simulink model "turnlamp"  (R2016a)
settings: Solver=ode1  StartTime=0.0  StopTime=Inf  FixedStep=0.001  RelTol=1e-3
PostLoadFcn:
  | , if any(exist('dsrtsu_mdlpostloadfcn', 'file') == [2, 3, 6]), try dsrtsu_mdlpostloadfcn('Execute', bdroot); catch fprintf('Error in PostLoadFcn (dsrtsu_mdlpostloadfcn) for model "%s":\n %s\n', bdroot, lasterr); end, end,
  | 
  | % Begin Version: 1.0
  | if(3 == exist('DSWatchDog')), DSWatchDog('OpenModel', get_param(bdroot(gcs),'filename')); end; assignin('base', sprintf('DS_%s_STATE', upper(bdroot(gcs))), 0);
  | % End Version: 1.0
StartFcn:
  | % Begin Version: 1.0
  | if(3 == exist('DSWatchDog')), DSWatchDog('StartModel', get_param(bdroot(gcs),'filename')); end; assignin('base', sprintf('DS_%s_STATE', upper(bdroot(gcs))), 2);
  | % End Version: 1.0
StopFcn:
  | % Begin Version: 1.0
  | if(3 == exist('DSWatchDog')), DSWatchDog('StopModel', get_param(bdroot(gcs),'filename')); end; assignin('base', sprintf('DS_%s_STATE', upper(bdroot(gcs))), 0);
  | % End Version: 1.0
libraries: simulink x2, simulink_extras x2
PreSaveFcn:
  | % Begin Version: 1.0
  | OldName = get_param(bdroot(gcs), 'Tag'); NewName = get_param(bdroot(gcs), 'filename'); if (~strcmp(OldName, NewName)), if(3 == exist('DSWatchDog')), DSWatchDog('CloseModel', OldName); DSWatchDog('OpenModel', NewName); end; set_param(bdroot(gcs), 'Tag', NewName); end; try, evalin('base', 'clear OldName NewName'); catch, disp('Error during execution of PreSaveFcn callback'); end;
  | % End Version: 1.0
PostSaveFcn:
  | % Begin Version: 1.0
  | if(3 == exist('DSWatchDog')), DSWatchDog('SaveModel', get_param(bdroot(gcs),'filename')); end;
  | % End Version: 1.0
CloseFcn:
  | % Begin Version: 1.0
  | if(3 == exist('DSWatchDog')), DSWatchDog('CloseModel', get_param(bdroot(gcs),'filename')); end; try, DS_STATE_NAME = sprintf('DS_%s_STATE', upper(bdroot(gcs))); evalin('base', 'clear(DS_STATE_NAME)'); evalin('base', 'clear DS_STATE_NAME'); catch, disp('Error during execution of CloseFcn callback'); end;
  | % End Version: 1.0
settings Model: Tag=C:\Users\Admin\Documents\dSPACE\Real-Time Testing\3.3\SampleExperiments\TurnSignal_VEOS\Model\turnlamp.slx  RTICANMMDATA=struct('GeneralSetupData',struct('modelroot',['C:\Users\Admin\Documents\dSPACE\Real-Time Testing\2.6\SampleExperiments\TurnSignal_VEOS\Model'],'generalsettings',struct('filesettings',struct('destfolder',struct('Name','RTICANMM_FILES','Check',1),'buildfolder',struct('Name','.','Check',1),'AbsDestfolder',struct('Name',['C:\Users\Admin\Documents\dSPACE\Real-Time Testing\2.6\SampleExperiments\TurnSignal_VEOS\Model\RTICANMM_FILES']),'AbsBuildfolder',struct('Name',['C:\Users\Admin\Documents\dSPACE\Real-Time Testing\2.6\SampleExperiments\TurnSignal_VEOS\Model']))),'options',struct('addpaths',1,'rmpaths',1,'addtrcexclusion',logical(1),'cannavigator',struct('checkmonitoring',0),'show_usrtrc',0,'use_usrtrc',0),'advanced',struct('options',[1 1 1 1 1 1 1 1 1 1 1 1 1 1 1 1 1 1 1 1 1 1 1 1 1 1 1 1 1 1 1 1 1 1 1 1 1 1 1 1 1 1 1 1 1 1 1 1 1 1 1 1 1 1 1 1 1 1 1 1 1 1 1 1 1 1 1 1 1 1 1 1 1 1 1 1 1 1 1 1 1 1 1 1 1 1 1 1 1 1 1 1 1 1 1 1 1 1 1 1]),'MPSetup',{{}},'modelname','turnlamp','block','turnlamp'))  RTILINMMDATA=struct('GeneralSetupData',[])  DSRTSU_INTERNAL_RTI_VER=460  DSRTSU_INTERNAL_RTI_TYPE=rti1401  DSRTSU_INTERNAL_RTIFLEXRAYCONFIG=80  DSRTSU_INTERNAL_RTIFPGA=50  ModifiedByFormat=dSPACE GmbH  ExtModeTrigMode=oneshot  ExtModeArmWhenConnect=off  Creator=dSPACE GmbH  LastModifiedBy=dSPACE GmbH
settings DataIOCC: LimitDataPoints=on  SaveFormat=Array  SignalLoggingSaveFormat=ModelDataLogs
settings OptimizationCC: BlockReduction=off  ConditionallyExecuteInputs=off  OptimizeBlockIOStorage=off  BufferReuse=off  GlobalBufferReuse=off  ExpressionFolding=off  ExpressionDepthLimit=2147483647  LocalBlockOutputs=off  InitFltsAndDblsToZero=on
settings DebuggingCC: SaveWithParameterizedLinksMsg=none  UnderspecifiedInitializationDetection=Classic  MergeDetectMultiDrivingBlocksExec=none  SignalResolutionControl=TryResolveAllWithWarning  MultiTaskDSMMsg=warning  MultiTaskCondExecSysMsg=none  MultiTaskRateTransMsg=warning  FcnCallInpInsideContextMsg=UseLocalSettings  StateNameClashWarn=warning
settings HardwareCC: ProdBitPerPointer=32  ProdLargestAtomicFloat=None  ProdIntDivRoundTo=Undefined  ProdEndianess=Unspecified  ProdWordSize=32  ProdHWDeviceType=32-bit Generic  TargetIntDivRoundTo=Zero  TargetEndianess=BigEndian  TargetHWDeviceType=Generic->Custom
settings ModelReferenceCC: PropagateSignalLabelsOutOfModel=off
settings RTWCC: SystemTargetFile=dsrt.tlc  GenCodeOnly=on  MakeCommand=make_dsrt  TemplateMakefile=dsrt_default_tmf  Description=dSPACE Run-Time Target  RTWVerbose=off
settings STFCustomTargetCC: ParMdlRefBuildCompliant=on  GeneratePreprocessorConditionals=Disable all  SystemTargetFile=dsrt.tlc
settings GRTTargetCC: CompOptLevelCompliant=off  ConcurrentExecutionCompliant=off  CombineOutputUpdateFcns=off  MatFileLogging=off  CPPClassGenCompliant=off  GRTInterface=on  UseToolchainInfoCompliant=off
settings ConfigComp: CovModelRefEnable=Off  CovSFcnEnable=off

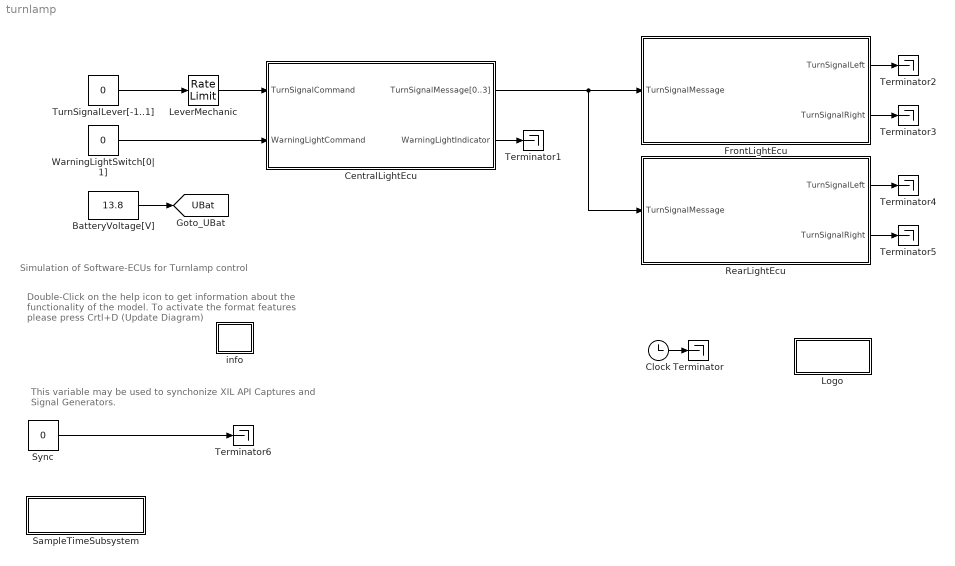
== system turnlamp ==
  note: This variable may be used to synchonize XIL API Captures
      | and Signal Generators.
  note: Simulation of Software-ECUs for Turnlamp control
  note: Double-Click on the help icon to get information about
      | the functionality of the model.
      |
      | To activate the format features please
      | press Crtl+D (Update Diagram)
  BatteryVoltage[V] : Constant  Value=13.8
  CentralLightEcu : Subsystem
  Clock : Clock
  FrontLightEcu : Subsystem
  LeverMechanic : RateLimiter  RisingSlewLimit=25  FallingSlewLimit=-25
  Logo : Subsystem  mask(dSPACE){EmptyParameter=[]}
      mask prompts: EmptyParameter "Mask Parameter 1:"
      settings: OpenFcn=;
      mask Display: image(imread('rti_mdl_dslogo.tif'));
  RearLightEcu : Subsystem
  SampleTimeSubsystem : Subsystem  TreatAsAtomicUnit=on  SystemSampleTime=0.01
  Sync : Constant  Value=0
  Terminator{,1..6} (7 alike) : Terminator
  TurnSignalLever[-1..1] : Constant  Value=0
  WarningLightSwitch[0|1] : Constant  Value=0
  info : Subsystem
      mask Display: disp('?')
  tag scope: UBat=global
  wires:
  TurnSignalLever[-1..1]/1 -> LeverMechanic/1
  LeverMechanic/1 -> CentralLightEcu/1(TurnSignalCommand)
  WarningLightSwitch[0|1]/1 -> CentralLightEcu/2(WarningLightCommand)
  CentralLightEcu/1(TurnSignalMessage[0..3]) -> FrontLightEcu/1(TurnSignalMessage), RearLightEcu/1(TurnSignalMessage)
  CentralLightEcu/2(WarningLightIndicator) -> Terminator1/1
  BatteryVoltage[V]/1 -> [UBat]
  FrontLightEcu/1(TurnSignalLeft) -> Terminator2/1
  FrontLightEcu/2(TurnSignalRight) -> Terminator3/1
  RearLightEcu/1(TurnSignalLeft) -> Terminator4/1
  RearLightEcu/2(TurnSignalRight) -> Terminator5/1
  Clock/1 -> Terminator/1
  Sync/1 -> Terminator6/1

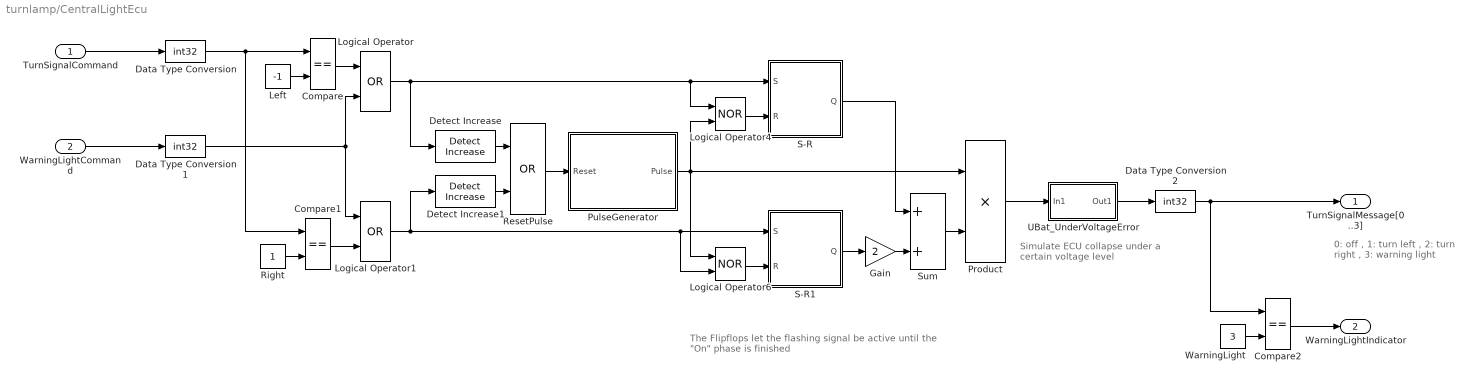
== system turnlamp/CentralLightEcu ==
  note: 0: off               ,
      | 1: turn left       ,
      | 2: turn right     ,
      | 3: warning light
  note: Simulate ECU collapse
      | under a certain voltage level
  note: The Flipflops let the flashing signal be active until
      | the "On" phase is finished
  TurnSignalCommand : Inport
  WarningLightCommand : Inport  Port=2
  Compare : RelationalOperator  Operator===  OutDataTypeStr=uint(8)  ZeroCross=off  InputSameDT=on
  Compare1 : RelationalOperator  Operator===  OutDataTypeStr=uint(8)  ZeroCross=off  InputSameDT=on
  Compare2 : RelationalOperator  Operator===  OutDataTypeStr=uint(8)  ZeroCross=off  InputSameDT=on
  Data Type Conversion : DataTypeConversion  OutDataTypeStr=int32  RndMeth=Zero
  Data Type Conversion1 : DataTypeConversion  OutDataTypeStr=int32  RndMeth=Zero
  Data Type Conversion2 : DataTypeConversion  OutDataTypeStr=int32  RndMeth=Zero
  Detect Increase : simulink/Logic and Bit Operations/Detect Increase  vinit=0.0  InputProcessing=Inherited  OutDataTypeStr=boolean
  Detect Increase1 : simulink/Logic and Bit Operations/Detect Increase  vinit=0.0  InputProcessing=Inherited  OutDataTypeStr=boolean
  Gain : Gain  Gain=2
  Left : Constant  Value=-1  OutDataTypeStr=Inherit: Inherit via back propagation
  Logical Operator : Logic  Operator=OR  AllPortsSameDT=off  OutDataTypeStr=uint(8)
  Logical Operator1 : Logic  Operator=OR  AllPortsSameDT=off  OutDataTypeStr=uint(8)
  Logical Operator4 : Logic  Operator=NOR  AllPortsSameDT=off  OutDataTypeStr=uint(8)
  Logical Operator6 : Logic  Operator=NOR  AllPortsSameDT=off  OutDataTypeStr=uint(8)
  Product : Product  RndMeth=Zero
  PulseGenerator : Subsystem
  ResetPulse : Logic  Operator=OR  AllPortsSameDT=off  OutDataTypeStr=uint(8)
  Right : Constant  OutDataTypeStr=Inherit: Inherit via back propagation
  S-R : Subsystem
  S-R1 : Subsystem
  Sum : Sum
  UBat_UnderVoltageError : Subsystem
  WarningLight : Constant  Value=3  OutDataTypeStr=Inherit: Inherit via back propagation
  TurnSignalMessage[0..3] : Outport
  WarningLightIndicator : Outport  Port=2
  wires:
  Data Type Conversion/1 -> Compare/1, Compare1/1
  Compare/1 -> Logical Operator/1
  Data Type Conversion1/1 -> Logical Operator/2, Logical Operator1/1
  Compare1/1 -> Logical Operator1/2
  Gain/1 -> Sum/2
  TurnSignalCommand/1 -> Data Type Conversion/1
  Product/1 -> UBat_UnderVoltageError/1(In1)
  WarningLightCommand/1 -> Data Type Conversion1/1
  Compare2/1 -> WarningLightIndicator/1
  Logical Operator/1 -> Logical Operator4/1, S-R/1(S), Detect Increase/1
  Logical Operator4/1 -> S-R/2(R)
  Logical Operator6/1 -> S-R1/2(R)
  Logical Operator1/1 -> Detect Increase1/1, Logical Operator6/2, S-R1/1(S)
  Detect Increase/1 -> ResetPulse/1
  Detect Increase1/1 -> ResetPulse/2
  ResetPulse/1 -> PulseGenerator/1(Reset)
  PulseGenerator/1(Pulse) -> Logical Operator4/2, Logical Operator6/1, Product/1
  Sum/1 -> Product/2
  S-R1/1(Q) -> Gain/1
  S-R/1(Q) -> Sum/1
  UBat_UnderVoltageError/1(Out1) -> Data Type Conversion2/1
  Data Type Conversion2/1 -> TurnSignalMessage[0..3]/1, Compare2/1
  Left/1 -> Compare/2
  Right/1 -> Compare1/2
  WarningLight/1 -> Compare2/2

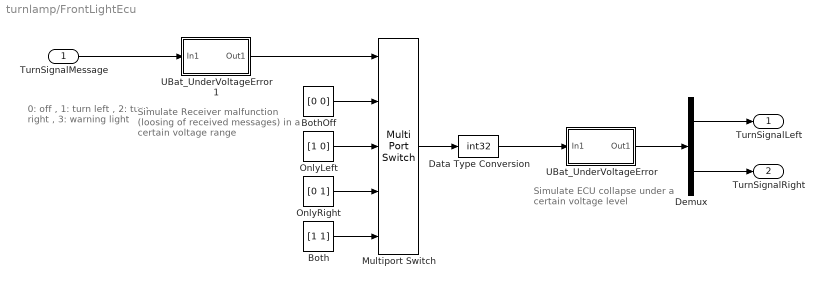
== system turnlamp/FrontLightEcu ==
  note: 0: off               ,
      | 1: turn left       ,
      | 2: turn right     ,
      | 3: warning light
  note: Simulate ECU collapse
      | under a certain voltage level
  note: Simulate Receiver malfunction
      | (loosing of received messages)
      | in a certain voltage range
  TurnSignalMessage : Inport
  Both : Constant  Value=[1 1]
  BothOff : Constant  Value=[0 0]
  Data Type Conversion : DataTypeConversion  OutDataTypeStr=int32  RndMeth=Zero
  Demux : Demux  Outputs=2
  Multiport Switch : MultiPortSwitch  DataPortOrder=Zero-based contiguous  Inputs=4  zeroidx=on
  OnlyLeft : Constant  Value=[1 0]
  OnlyRight : Constant  Value=[0 1]
  UBat_UnderVoltageError : Subsystem
  UBat_UnderVoltageError1 : Subsystem
  TurnSignalLeft : Outport
  TurnSignalRight : Outport  Port=2
  wires:
  TurnSignalMessage/1 -> UBat_UnderVoltageError1/1(In1)
  BothOff/1 -> Multiport Switch/2
  OnlyLeft/1 -> Multiport Switch/3
  OnlyRight/1 -> Multiport Switch/4
  Both/1 -> Multiport Switch/5
  Multiport Switch/1 -> Data Type Conversion/1
  Data Type Conversion/1 -> UBat_UnderVoltageError/1(In1)
  UBat_UnderVoltageError/1(Out1) -> Demux/1
  Demux/1 -> TurnSignalLeft/1
  Demux/2 -> TurnSignalRight/1
  UBat_UnderVoltageError1/1(Out1) -> Multiport Switch/1

== system turnlamp/Logo ==
  note: $Revision: 1.3 $
  note: $Date: 2009/04/30 09:39:12GMT+01:00 $
  note: $Workfile: smd_1006_sl.mdl $

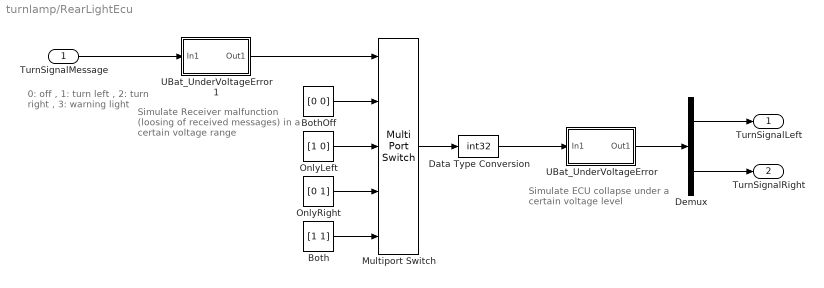
== system turnlamp/RearLightEcu ==
  note: 0: off               ,
      | 1: turn left       ,
      | 2: turn right     ,
      | 3: warning light
  note: Simulate Receiver malfunction
      | (loosing of received messages)
      | in a certain voltage range
  note: Simulate ECU collapse
      | under a certain voltage level
  TurnSignalMessage : Inport
  Both : Constant  Value=[1 1]
  BothOff : Constant  Value=[0 0]
  Data Type Conversion : DataTypeConversion  OutDataTypeStr=int32  RndMeth=Zero
  Demux : Demux  Outputs=2
  Multiport Switch : MultiPortSwitch  DataPortOrder=Zero-based contiguous  Inputs=4  zeroidx=on
  OnlyLeft : Constant  Value=[1 0]
  OnlyRight : Constant  Value=[0 1]
  UBat_UnderVoltageError : Subsystem
  UBat_UnderVoltageError1 : Subsystem
  TurnSignalLeft : Outport
  TurnSignalRight : Outport  Port=2
  wires:
  UBat_UnderVoltageError1/1(Out1) -> Multiport Switch/1
  Demux/2 -> TurnSignalRight/1
  Demux/1 -> TurnSignalLeft/1
  UBat_UnderVoltageError/1(Out1) -> Demux/1
  Data Type Conversion/1 -> UBat_UnderVoltageError/1(In1)
  Multiport Switch/1 -> Data Type Conversion/1
  Both/1 -> Multiport Switch/5
  OnlyRight/1 -> Multiport Switch/4
  OnlyLeft/1 -> Multiport Switch/3
  BothOff/1 -> Multiport Switch/2
  TurnSignalMessage/1 -> UBat_UnderVoltageError1/1(In1)

== system turnlamp/SampleTimeSubsystem ==
  A1 : Constant  Value=0
  Terminator5 : Terminator
  info : Subsystem
      mask Display: disp('?')
  wires:
  A1/1 -> Terminator5/1

== system turnlamp/info ==
  note: .
  note: This model simulates the behaviour of three ECUs for controlling TurnSignals,
      | dependent on a TurnSignalLever and a WarningLightSwitch
  note: Aim of this demo: to show possibilities of different ECU test procedures
  note: To control this model, use the corresponding ControlDesk experiment:
      | - Set TurnSignalLever to Left, Right or Off
      | - Switch WarningLight Switch to Off or On
      | - Change the Battery voltage: below a certain voltage level, some (simulated) malfunctions may occur
      |    - <= 7.2V, the ECUs will collapse completely
      |    - <= 8.2 V (dependent on voltage, more effect with lower voltage), simulated receiver in front and rear ECU become unstable,
      |      thus the timing of the generated TurnSignal will be disturbed

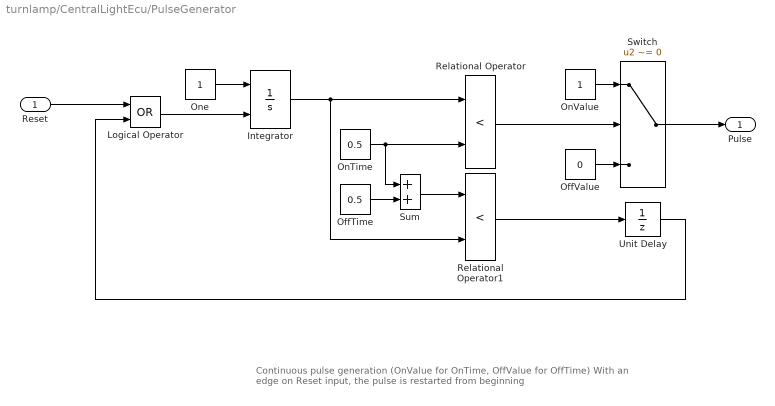
== system turnlamp/CentralLightEcu/PulseGenerator ==
  note: Continuous pulse generation (OnValue for OnTime, OffValue for OffTime)
      | With an edge on Reset input, the pulse is restarted from beginning
  Reset : Inport
  Integrator : Integrator  ExternalReset=rising
  Logical Operator : Logic  Operator=OR  AllPortsSameDT=off  OutDataTypeStr=boolean
  OffTime : Constant  Value=0.5
  OffValue : Constant  Value=0
  OnTime : Constant  Value=0.5
  OnValue : Constant
  One : Constant
  Relational Operator : RelationalOperator  Operator=<  OutDataTypeStr=boolean
  Relational Operator1 : RelationalOperator  Operator=<  OutDataTypeStr=boolean
  Sum : Sum
  Switch : Switch  Criteria=u2 ~= 0
  Unit Delay : UnitDelay  SampleTime=-1
  Pulse : Outport
  wires:
  Switch/1 -> Pulse/1
  Integrator/1 -> Relational Operator/1, Relational Operator1/2
  OnTime/1 -> Relational Operator/2, Sum/1
  Relational Operator/1 -> Switch/2
  OnValue/1 -> Switch/1
  OffValue/1 -> Switch/3
  One/1 -> Integrator/1
  OffTime/1 -> Sum/2
  Sum/1 -> Relational Operator1/1
  Relational Operator1/1 -> Unit Delay/1
  Logical Operator/1 -> Integrator/2
  Reset/1 -> Logical Operator/1
  Unit Delay/1 -> Logical Operator/2

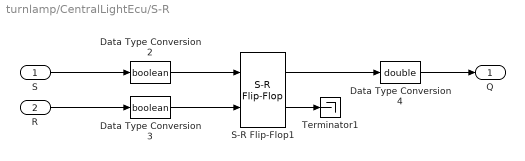
== system turnlamp/CentralLightEcu/S-R ==
  S : Inport
  R : Inport  Port=2
  Data Type Conversion2 : DataTypeConversion  OutDataTypeStr=boolean  RndMeth=Zero
  Data Type Conversion3 : DataTypeConversion  OutDataTypeStr=boolean  RndMeth=Zero
  Data Type Conversion4 : DataTypeConversion  OutDataTypeStr=double  RndMeth=Zero
  S-R Flip-Flop1 : simulink_extras/Flip Flops/S-R Flip-Flop  initial_condition=0
  Terminator1 : Terminator
  Q : Outport
  wires:
  R/1 -> Data Type Conversion3/1
  Data Type Conversion4/1 -> Q/1
  S/1 -> Data Type Conversion2/1
  S-R Flip-Flop1/1 -> Data Type Conversion4/1
  Data Type Conversion3/1 -> S-R Flip-Flop1/2
  Data Type Conversion2/1 -> S-R Flip-Flop1/1
  S-R Flip-Flop1/2 -> Terminator1/1

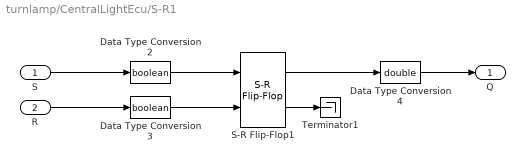
== system turnlamp/CentralLightEcu/S-R1 ==
  S : Inport
  R : Inport  Port=2
  Data Type Conversion2 : DataTypeConversion  OutDataTypeStr=boolean  RndMeth=Zero
  Data Type Conversion3 : DataTypeConversion  OutDataTypeStr=boolean  RndMeth=Zero
  Data Type Conversion4 : DataTypeConversion  OutDataTypeStr=double  RndMeth=Zero
  S-R Flip-Flop1 : simulink_extras/Flip Flops/S-R Flip-Flop  initial_condition=0
  Terminator1 : Terminator
  Q : Outport
  wires:
  S-R Flip-Flop1/2 -> Terminator1/1
  Data Type Conversion2/1 -> S-R Flip-Flop1/1
  Data Type Conversion3/1 -> S-R Flip-Flop1/2
  S-R Flip-Flop1/1 -> Data Type Conversion4/1
  S/1 -> Data Type Conversion2/1
  Data Type Conversion4/1 -> Q/1
  R/1 -> Data Type Conversion3/1

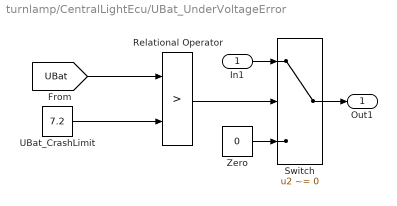
== system turnlamp/CentralLightEcu/UBat_UnderVoltageError ==
  In1 : Inport
  Relational Operator : RelationalOperator  Operator=>  OutDataTypeStr=boolean
  Switch : Switch  Criteria=u2 ~= 0
  UBat_CrashLimit : Constant  Value=7.2
  Zero : Constant  Value=0
  Out1 : Outport
  wires:
  UBat_CrashLimit/1 -> Relational Operator/2
  [UBat] -> Relational Operator/1
  Relational Operator/1 -> Switch/2
  Zero/1 -> Switch/3
  In1/1 -> Switch/1
  Switch/1 -> Out1/1

== system turnlamp/FrontLightEcu/UBat_UnderVoltageError ==
  In1 : Inport
  Relational Operator : RelationalOperator  Operator=>  OutDataTypeStr=boolean
  Switch : Switch  Criteria=u2 ~= 0
  UBat_CrashLimit : Constant  Value=7.2
  Zero : Constant  Value=0
  Out1 : Outport
  wires:
  Switch/1 -> Out1/1
  In1/1 -> Switch/1
  Zero/1 -> Switch/3
  Relational Operator/1 -> Switch/2
  [UBat] -> Relational Operator/1
  UBat_CrashLimit/1 -> Relational Operator/2

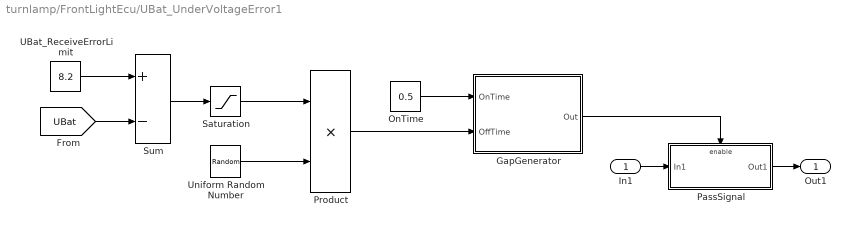
== system turnlamp/FrontLightEcu/UBat_UnderVoltageError1 ==
  In1 : Inport
  GapGenerator : Subsystem
  OnTime : Constant  Value=0.5
  PassSignal : Subsystem  TreatAsAtomicUnit=on
  Product : Product  RndMeth=Zero
  Saturation : Saturate  UpperLimit=1.2  LowerLimit=0.0
  Sum : Sum  Inputs=+-
  UBat_ReceiveErrorLimit : Constant  Value=8.2
  Uniform Random Number : UniformRandomNumber  Minimum=0  SampleTime=0
  Out1 : Outport
  wires:
  In1/1 -> PassSignal/1(In1)
  PassSignal/1(Out1) -> Out1/1
  GapGenerator/1(Out) -> PassSignal/Enable
  OnTime/1 -> GapGenerator/1(OnTime)
  Sum/1 -> Saturation/1
  UBat_ReceiveErrorLimit/1 -> Sum/1
  [UBat] -> Sum/2
  Saturation/1 -> Product/1
  Product/1 -> GapGenerator/2(OffTime)
  Uniform Random Number/1 -> Product/2

== system turnlamp/RearLightEcu/UBat_UnderVoltageError ==
  In1 : Inport
  Relational Operator : RelationalOperator  Operator=>  OutDataTypeStr=boolean
  Switch : Switch  Criteria=u2 ~= 0
  UBat_CrashLimit : Constant  Value=7.2
  Zero : Constant  Value=0
  Out1 : Outport
  wires:
  UBat_CrashLimit/1 -> Relational Operator/2
  [UBat] -> Relational Operator/1
  Relational Operator/1 -> Switch/2
  Zero/1 -> Switch/3
  In1/1 -> Switch/1
  Switch/1 -> Out1/1

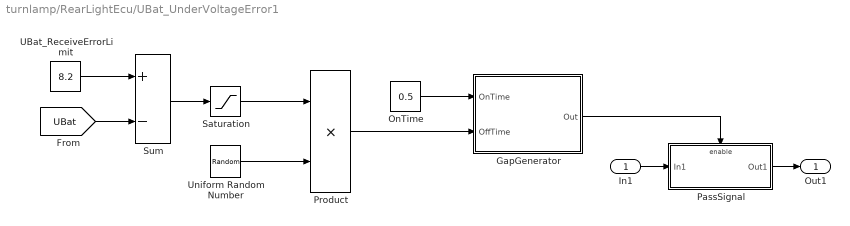
== system turnlamp/RearLightEcu/UBat_UnderVoltageError1 ==
  In1 : Inport
  GapGenerator : Subsystem
  OnTime : Constant  Value=0.5
  PassSignal : Subsystem  TreatAsAtomicUnit=on
  Product : Product  RndMeth=Zero
  Saturation : Saturate  UpperLimit=1.2  LowerLimit=0.0
  Sum : Sum  Inputs=+-
  UBat_ReceiveErrorLimit : Constant  Value=8.2
  Uniform Random Number : UniformRandomNumber  Minimum=0  Seed=1  SampleTime=0
  Out1 : Outport
  wires:
  Uniform Random Number/1 -> Product/2
  Product/1 -> GapGenerator/2(OffTime)
  Saturation/1 -> Product/1
  [UBat] -> Sum/2
  UBat_ReceiveErrorLimit/1 -> Sum/1
  Sum/1 -> Saturation/1
  OnTime/1 -> GapGenerator/1(OnTime)
  GapGenerator/1(Out) -> PassSignal/Enable
  PassSignal/1(Out1) -> Out1/1
  In1/1 -> PassSignal/1(In1)

== system turnlamp/SampleTimeSubsystem/info ==
  note: .
  note: This subsystems realizes a new sampling period for measurements. It is configured with a step size of 10 ms.

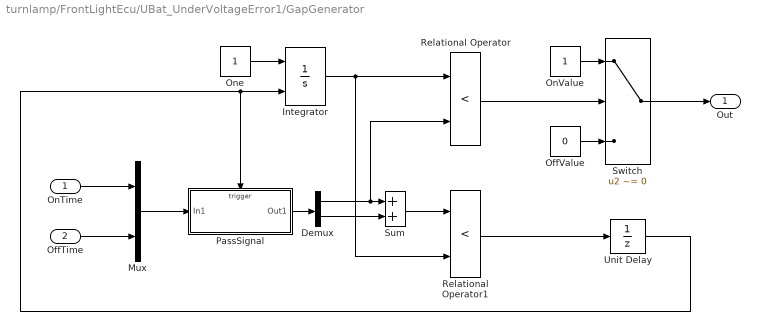
== system turnlamp/FrontLightEcu/UBat_UnderVoltageError1/GapGenerator ==
  OnTime : Inport
  OffTime : Inport  Port=2
  Demux : Demux  Outputs=2
  Integrator : Integrator  ExternalReset=rising
  Mux : Mux  Inputs=2
  OffValue : Constant  Value=0
  OnValue : Constant
  One : Constant
  PassSignal : Subsystem  TreatAsAtomicUnit=on
  Relational Operator : RelationalOperator  Operator=<  OutDataTypeStr=boolean
  Relational Operator1 : RelationalOperator  Operator=<  OutDataTypeStr=boolean
  Sum : Sum
  Switch : Switch  Criteria=u2 ~= 0
  Unit Delay : UnitDelay  InitialCondition=1  SampleTime=-1
  Out : Outport
  wires:
  Switch/1 -> Out/1
  Integrator/1 -> Relational Operator/1, Relational Operator1/2
  Relational Operator/1 -> Switch/2
  OnValue/1 -> Switch/1
  OffValue/1 -> Switch/3
  One/1 -> Integrator/1
  Sum/1 -> Relational Operator1/1
  Relational Operator1/1 -> Unit Delay/1
  Unit Delay/1 -> Integrator/2, PassSignal/Trigger
  Demux/1 -> Relational Operator/2, Sum/1
  Demux/2 -> Sum/2
  PassSignal/1(Out1) -> Demux/1
  Mux/1 -> PassSignal/1(In1)
  OnTime/1 -> Mux/1
  OffTime/1 -> Mux/2

== system turnlamp/FrontLightEcu/UBat_UnderVoltageError1/PassSignal ==
  In1 : Inport
  Enable : EnablePort
  Data Type Conversion2 : DataTypeConversion  RndMeth=Zero
  Out1 : Outport  InitialOutput=[0]
  wires:
  In1/1 -> Data Type Conversion2/1
  Data Type Conversion2/1 -> Out1/1

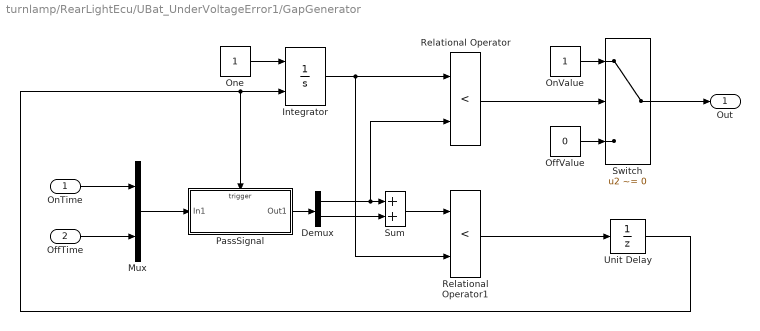
== system turnlamp/RearLightEcu/UBat_UnderVoltageError1/GapGenerator ==
  OnTime : Inport
  OffTime : Inport  Port=2
  Demux : Demux  Outputs=2
  Integrator : Integrator  ExternalReset=rising
  Mux : Mux  Inputs=2
  OffValue : Constant  Value=0
  OnValue : Constant
  One : Constant
  PassSignal : Subsystem  TreatAsAtomicUnit=on
  Relational Operator : RelationalOperator  Operator=<  OutDataTypeStr=boolean
  Relational Operator1 : RelationalOperator  Operator=<  OutDataTypeStr=boolean
  Sum : Sum
  Switch : Switch  Criteria=u2 ~= 0
  Unit Delay : UnitDelay  InitialCondition=1  SampleTime=-1
  Out : Outport
  wires:
  OffTime/1 -> Mux/2
  OnTime/1 -> Mux/1
  Mux/1 -> PassSignal/1(In1)
  PassSignal/1(Out1) -> Demux/1
  Demux/2 -> Sum/2
  Demux/1 -> Sum/1, Relational Operator/2
  Unit Delay/1 -> PassSignal/Trigger, Integrator/2
  Relational Operator1/1 -> Unit Delay/1
  Sum/1 -> Relational Operator1/1
  One/1 -> Integrator/1
  OffValue/1 -> Switch/3
  OnValue/1 -> Switch/1
  Relational Operator/1 -> Switch/2
  Integrator/1 -> Relational Operator1/2, Relational Operator/1
  Switch/1 -> Out/1

== system turnlamp/RearLightEcu/UBat_UnderVoltageError1/PassSignal ==
  In1 : Inport
  Enable : EnablePort
  Data Type Conversion2 : DataTypeConversion  RndMeth=Zero
  Out1 : Outport  InitialOutput=[0]
  wires:
  Data Type Conversion2/1 -> Out1/1
  In1/1 -> Data Type Conversion2/1

== system turnlamp/FrontLightEcu/UBat_UnderVoltageError1/GapGenerator/PassSignal ==
  In1 : Inport
  Trigger : TriggerPort  VariantControl=Variant
  Gain : Gain
  Out1 : Outport  InitialOutput=[0.5 0]
  wires:
  In1/1 -> Gain/1
  Gain/1 -> Out1/1

== system turnlamp/RearLightEcu/UBat_UnderVoltageError1/GapGenerator/PassSignal ==
  In1 : Inport
  Trigger : TriggerPort  VariantControl=Variant
  Gain : Gain
  Out1 : Outport  InitialOutput=[0.5 0]
  wires:
  Gain/1 -> Out1/1
  In1/1 -> Gain/1
